simulink model "Preleva1"  (R2019a)
settings: Solver=VariableStepAuto  StartTime=0.0  StopTime=10.0  RelTol=1e-3
settings Model: Creator=anton  LastModifiedBy=anton

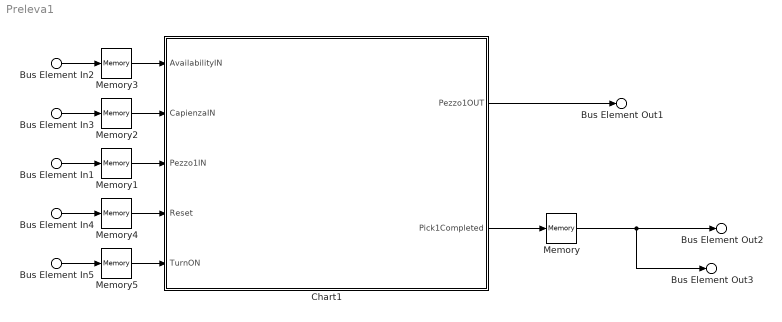
== system Preleva1 ==
  Bus Element In1 : Inport  PortName=Pezzo1
  Bus Element In2 : Inport  Port=2  PortName=AvailabilityIN
  Bus Element In4 : Inport  Port=3  PortName=Reset
  Bus Element In5 : Inport  Port=4  PortName=TurnON
  Bus Element In3 : Inport  Port=5  PortName=CapienzaIN
  Chart1 : Stateflow chart  BlockKeywords=__PRM__SERIALIZED__DATA__:Stateflow Chart,Stateflow Diagram  TreatAsAtomicUnit=on
  Memory{,1..5} (6 alike) : Memory
  Bus Element Out1 : Outport  PortName=Pezzo1OUT
  Bus Element Out3 : Outport  Port=2  PortName=Pick1CompletedOUT
  Bus Element Out2 : Outport  Port=3  PortName=Pick1Completed
  wires:
  Chart1/1(Pezzo1OUT) -> Bus Element Out1/1
  Chart1/2(Pick1Completed) -> Memory/1
  Memory/1 -> Bus Element Out3/1, Bus Element Out2/1
  Bus Element In2/1 -> Memory3/1
  Memory3/1 -> Chart1/1(AvailabilityIN)
  Bus Element In3/1 -> Memory2/1
  Memory2/1 -> Chart1/2(CapienzaIN)
  Bus Element In1/1 -> Memory1/1
  Memory1/1 -> Chart1/3(Pezzo1IN)
  Bus Element In4/1 -> Memory4/1
  Memory4/1 -> Chart1/4(Reset)
  Bus Element In5/1 -> Memory5/1
  Memory5/1 -> Chart1/5(TurnON)

== stateflow chart Preleva1/Chart1 ==
  state Idle
    Pezzo1OUT=0;
    Pick1Completed=0;
  state Waiting
    Pezzo1OUT=0;
    Pick1Completed=0;
  state Active
  state Working
  state Place
    during:
    Pezzo1OUT=1;
    Pick1Completed = 1;
  state Pick
    pause(0.1);
  (default) -> Idle
  Place -> Idle [order 1] : [TurnON==0]
  Idle -> Active : [TurnON==1]
  Waiting -> Idle [order 2] : [TurnON==0]
  Pick -> Idle [order 2] : [TurnON==0]
  Working -> Idle [order 2] : [TurnON==0]
  Active -> Working
  Place -> Waiting [order 2] : [after(1,sec)]
  Waiting -> Working [order 1] : [Reset==1]
  Working -> Pick [order 1] : [AvailabilityIN==1 && CapienzaIN>0 && Pezzo1IN==1]
  Pick -> Place [order 1] : [after(10,sec)]
  data: AvailabilityIN input; CapienzaIN input; Pezzo1IN input; Pezzo1OUT output; Pick1Completed output; Reset input; TurnON input
